simulink model "untitled1"  (R2025a)
settings: Solver=FixedStepAuto  StartTime=0.0  StopTime=0.5  FixedStep=1e-5  RelTol=1e-3
settings Model: Creator=jekir  LastModifiedBy=jekir

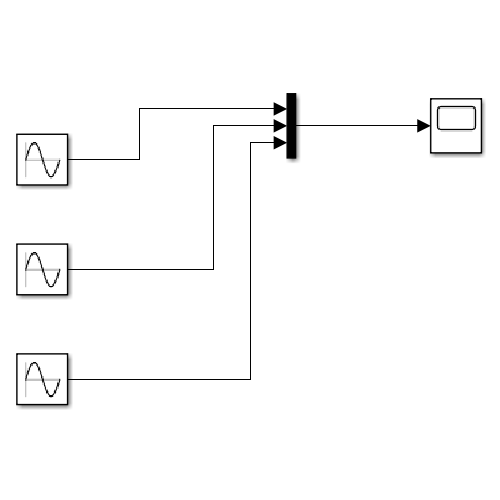
[thumbnail: Simulink's stored preview of the top-level diagram]
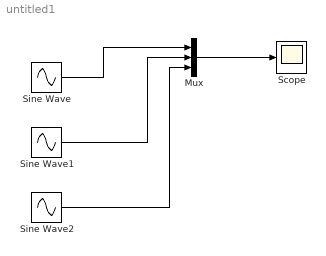
== system untitled1 ==
  Mux : Mux  Inputs=3
  Scope : Scope
      settings: ActiveDisplayYMinimum=-1.3374229221525806  ActiveDisplayYMaximum=1.1943131967846781
  Sine Wave : Sin  Frequency=2*pi*50  SampleTime=0
  Sine Wave1 : Sin  Frequency=2*pi*50  Phase=-pi/3  SampleTime=0
  Sine Wave2 : Sin  Frequency=2*pi*50  Phase=pi/3  SampleTime=0
  wires:
  Sine Wave/1 -> Mux/1
  Mux/1 -> Scope/1
  Sine Wave1/1 -> Mux/2
  Sine Wave2/1 -> Mux/3
